simulink library "filteredPIDController_ul"  (R2018b)
settings: Solver=VariableStepAuto  StartTime=0.0  StopTime=10.0  RelTol=1e-3
undefined symbols (not defined in the file): tau
settings Model: Creator=mcobb  LastModifiedBy=mcobb

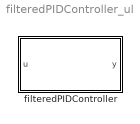
== system filteredPIDController_ul ==
  filteredPIDController : Subsystem  mask{kp=0, ki=0, kd=0, Parameter4=0}
      mask prompts: kp "Proportional Gain"; ki "Integral Gain"; kd "Derivative Gain"; Parameter4 "Filter Time Constant [s]"

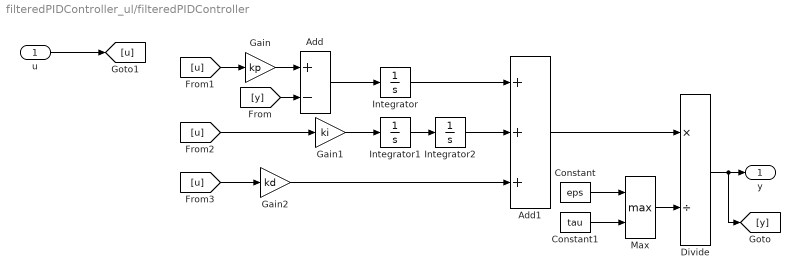
== system filteredPIDController_ul/filteredPIDController ==
  u : Inport
  Add : Sum  Inputs=+-
  Add1 : Sum  Inputs=+++
  Constant : Constant  Value=eps
  Constant1 : Constant  Value=tau
  Divide : Product  Inputs=*/
  Gain : Gain  Gain=kp
  Gain1 : Gain  Gain=ki
  Gain2 : Gain  Gain=kd
  Integrator : Integrator
  Integrator1 : Integrator
  Integrator2 : Integrator
  Max : MinMax  Function=max  Inputs=2
  y : Outport
  wires:
  u/1 -> [u]
  Gain/1 -> Add/1
  [y] -> Add/2
  Add/1 -> Integrator/1
  [u] -> Gain/1
  Max/1 -> Divide/2
  Constant/1 -> Max/1
  Constant1/1 -> Max/2
  Integrator1/1 -> Integrator2/1
  Gain1/1 -> Integrator1/1
  [u] -> Gain1/1
  [u] -> Gain2/1
  Integrator2/1 -> Add1/2
  Integrator/1 -> Add1/1
  Gain2/1 -> Add1/3
  Add1/1 -> Divide/1
  Divide/1 -> [y], y/1
